simulink library "cstextras"  (Simulink 7.1)
settings Model: Creator=greg  LastModifiedBy=pascal

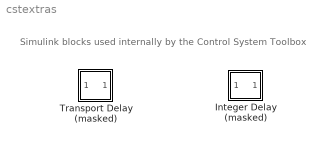
== system cstextras ==
  note: Simulink blocks used internally by
      | the Control System Toolbox
  Integer Delay (masked) : Subsystem  mask(Integer Delay (masked)){Td=1, u0=0, Ts=1}
      mask prompts: Td "Number of Delays"; u0 "Initial Input"; Ts "Sample Time"
      mask help: Integer Delay, with direct feedthrough when Delay Time is equal to zero.
      mask init:
      | str = '1/z^N';
      | df = get_param(bdroot,'dirty');
      | % Scalar expansion (do it here otherwise
      | % u0(j) and Td(j) settings in Integer
      | % Delay blocks are invalid and cause error)
      | if isscalar(u0), u0 = u0*ones(size(Td)); end
      | if isscalar(Td), Td = Td*ones(size(u0)); end
      | % Build reprsentation of delay vector
      | idfthru(gcb, Td, u0);
      | set_param(bdroot,'dirty',df)
      mask Help: See Integer Delay for more information.
      mask Display: block_icon('Integer Delay')
  Transport Delay (masked) : Subsystem  mask(Transport Delay (masked)){Td=1, u0=0, bufsize=1024}
      mask prompts: Td "Delay Time"; u0 "Initial Input"; bufsize "Initial Buffer Size"
      mask help: Transport Delay, with direct feedthrough when Delay Time is equal to zero.
      mask init:
      | df = get_param(bdroot,'dirty');
      | % Scalar expansion (do it here otherwise
      | % u0(j) and Td(j) settings in Transport
      | % Delay blocks are invalid and cause error)
      | if isscalar(u0), u0 = u0*ones(size(Td)); end
      | if isscalar(Td), Td = Td*ones(size(u0)); end
      | % Build reprsentation of delay vector
      | tdfthru(gcb, Td, u0, bufsize);
      | set_param(bdroot,'dirty',df)
      mask Help: See Transport Delay for more information.
      mask Display: block_icon('Transport Delay')

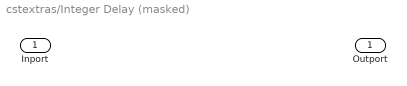
== system cstextras/Integer Delay (masked) ==
  Inport : Inport  OutDataType=sfix(16)  OutScaling=2^0
  Outport : Outport  OutDataType=sfix(16)  OutScaling=2^0

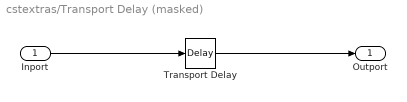
== system cstextras/Transport Delay (masked) ==
  Inport : Inport  OutDataType=sfix(16)  OutScaling=2^0
  Transport Delay : TransportDelay
  Outport : Outport  OutDataType=sfix(16)  OutScaling=2^0
  wires:
  Inport/1 -> Transport Delay/1
  Transport Delay/1 -> Outport/1
